simulink model "Robust_Adaptive_Control"  (R2015a)
settings: Solver=ode45  StartTime=0.0  StopTime=10  FixedStep=1e-3
libraries: aerolibutil x16, aerolibtransform2 x6, dspmtrx3 x6, simulink x1
(part 3 of 3)

== matlab function Robust_Adaptive_Control/y Gen./M(q),C(q,dq),g(q)_1/M,H/W6 ==
  data: w1 input; W output; w2 input; w3 input
function W = fcn(w1,w2,w3)

W = [0    -w3  w2
     w3  0    -w1
    -w2  w1  0];

== matlab function Robust_Adaptive_Control/y Gen./M(q),C(q,dq),g(q)_2/M,H/MATLAB Function ==
  data: m input; M output; I1 input; I2 input; I3 input; I4 input; I5 input; I6 input; W1 input; W2 input; W3 input; W4 input; W5 input; W6 input; H output
function [M,H] = fcn(m,I1,I2,I3,I4,I5,I6,W1,W2,W3,W4,W5,W6)
%#codegen

M = blkdiag(m(1)*eye(3),m(2)*eye(3),m(3)*eye(3),m(4)*eye(3),m(5)*eye(3),m(6)*eye(3),...
            I1,I2,I3,I4,I5,I6);

H =-blkdiag(zeros(18,18),W1,W2,W3,W4,W5,W6);

== matlab function Robust_Adaptive_Control/y Gen./M(q),C(q,dq),g(q)_2/M,H/W1 ==
  data: w1 input; W output; w2 input; w3 input
function W = fcn(w1,w2,w3)

W = [0    -w3  w2
     w3    0  -w1
    -w2    w1  0];

== matlab function Robust_Adaptive_Control/y Gen./M(q),C(q,dq),g(q)_2/M,H/W2 ==
  data: w1 input; W output; w2 input; w3 input
function W = fcn(w1,w2,w3)

W = [0    -w3  w2
     w3  0    -w1
    -w2  w1  0];

== matlab function Robust_Adaptive_Control/y Gen./M(q),C(q,dq),g(q)_2/M,H/W3 ==
  data: w1 input; W output; w2 input; w3 input
function W = fcn(w1,w2,w3)

W = [0    -w3  w2
     w3  0    -w1
    -w2  w1  0];

== matlab function Robust_Adaptive_Control/y Gen./M(q),C(q,dq),g(q)_2/M,H/W4 ==
  data: w1 input; W output; w2 input; w3 input
function W = fcn(w1,w2,w3)

W = [0    -w3  w2
     w3  0    -w1
    -w2  w1  0];

== matlab function Robust_Adaptive_Control/y Gen./M(q),C(q,dq),g(q)_2/M,H/W5 ==
  data: w1 input; W output; w2 input; w3 input
function W = fcn(w1,w2,w3)

W = [0    -w3  w2
     w3  0    -w1
    -w2  w1  0];

== matlab function Robust_Adaptive_Control/y Gen./M(q),C(q,dq),g(q)_2/M,H/W6 ==
  data: w1 input; W output; w2 input; w3 input
function W = fcn(w1,w2,w3)

W = [0    -w3  w2
     w3  0    -w1
    -w2  w1  0];

== matlab function Robust_Adaptive_Control/y Gen./MATLAB Function ==
  data: y1 input; y output; y2 input
function y = fcn(y1,y2)
%#codegen

y = [y1,y2];
